simulink model "chart"  (R2025b)
settings: Solver=VariableStepAuto  StartTime=0.0  StopTime=10.0  RelTol=1e-3
undefined symbols (not defined in the file or in its folder): AppAirBtn, AppAmplitude, AppPeriods, AppSharpness, AppZeroBtn, xx, yy
libraries: slrealtimeutilitieslib x7, dspstat3 x2, simulink x1, etargetslib x1, dspmathops x1
settings Model: Creator=Huawei  LastModifiedBy=Huawei

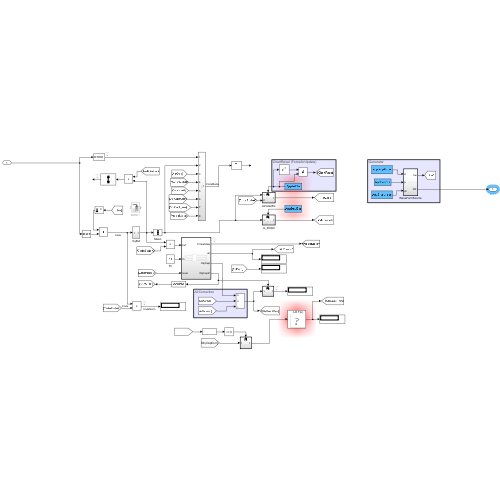
[thumbnail: Simulink's stored preview of the top-level diagram]
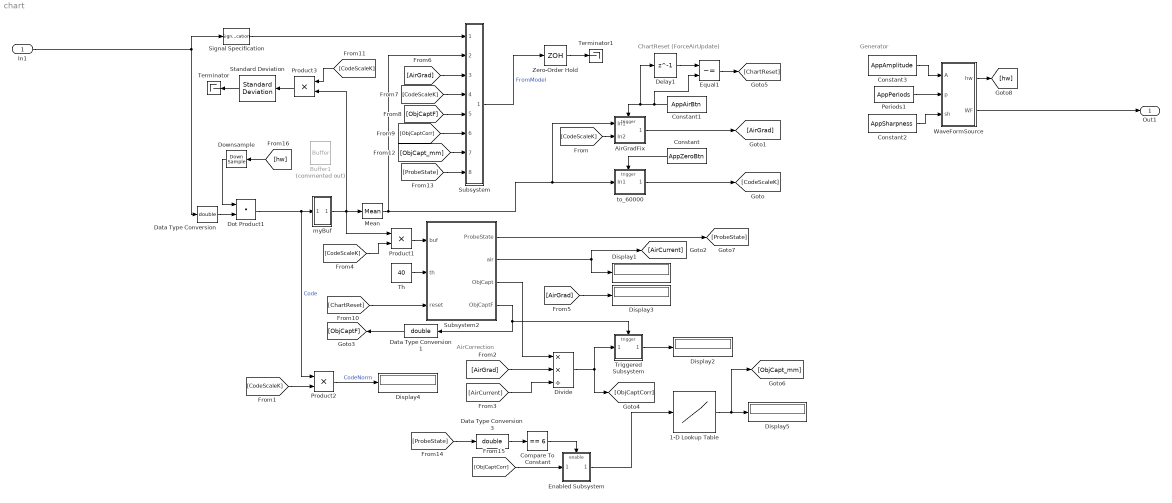
== system chart ==
  note: AirCorrection
  note: ChartReset (ForceAirUpdate)
  note: Generator
  In1 : Inport
  1-D Lookup Table : Lookup_n-D  NumberOfTableDimensions=1  LookupTableObject=myLUTobj  BreakpointsForDimension1=xx  IndexSearchMethod=Linear search  Table=yy  InternalRulePriority=Speed  RndMeth=Simplest
  AirGradFix : Subsystem  TreatAsAtomicUnit=on
  Buffer1 : Buffer  Commented=on  N=8  V=7  OutputFrames=off
  Compare To Constant : simulink/Logic and Bit Operations/Compare To Constant  relop===  const=6  OutDataTypeStr=boolean
  Constant : Constant  Value=AppZeroBtn  OutDataTypeStr=boolean  SampleTime=0.02
  Constant1 : Constant  Value=AppAirBtn  OutDataTypeStr=boolean  SampleTime=0.02
  Constant2 : Constant  Value=AppSharpness  SampleTime=0.02
  Constant3 : Constant  Value=AppAmplitude  SampleTime=0.02
  Data Type Conversion : DataTypeConversion  OutDataTypeStr=double  SaturateOnIntegerOverflow=off  RndMeth=Floor
  Data Type Conversion1 : DataTypeConversion  OutDataTypeStr=double  SaturateOnIntegerOverflow=off  RndMeth=Floor
  Data Type Conversion3 : DataTypeConversion  OutDataTypeStr=double  SaturateOnIntegerOverflow=off  RndMeth=Floor
  Delay1 : Delay  DelayLength=1  InputProcessing=Columns as channels (frame based)
  Display{1..5} (5 alike) : Display
      settings: Format=bank
  Divide : Product  Inputs=**/
  Dot Product1 : DotProduct  OutDataTypeStr=Inherit: Inherit via internal rule
  Downsample : DownSample  N=4
  Enabled Subsystem : Subsystem  TreatAsAtomicUnit=on
  Equal1 : RelationalOperator  Operator=~=  OutDataTypeStr=boolean  RndMeth=Simplest  InputSameDT=off
  Mean : dspstat3/Mean  run=off  InputProcessing=Columns as channels (frame based)  reset_popup=None  directionMode=Each column  dimension=1  roiEnable=off  roiType=Rectangles  roiPortion=Entire ROI  roiOutput=Individual statistics for each ROI  roiFlag=off  roundingMode=Floor  overflowMode=off  outputDataTypeStr=Inherit: Same as accumulator  outputMin=[]  outputMax=[]  outputLastDataTypeStr=Inherit: Same as accumulator
  Periods1 : Constant  Value=AppPeriods  SampleTime=0.02
  Product1 : Product
  Product2 : Product
  Product3 : Product
  Signal Specification : SignalSpecification  Dimensions=5000
  Standard Deviation : dspstat3/Standard Deviation  run=off  directionMode=Each column  dimension=1  InputProcessing=Columns as channels (frame based)  reset_popup=None  roiEnable=off  roiType=Rectangles  roiPortion=Entire ROI  roiOutput=Individual statistics for each ROI  roiFlag=off
  Subsystem : Subsystem
  Subsystem2 : Subsystem  TreatAsAtomicUnit=on  SystemSampleTime=0.02
  Terminator : Terminator
  Terminator1 : Terminator
  Th : Constant  Value=40  SampleTime=0.02
  Triggered Subsystem : Subsystem  TreatAsAtomicUnit=on
  WaveFormSource : Subsystem  TreatAsAtomicUnit=on  SystemSampleTime=0.02
  Zero-Order Hold : ZeroOrderHold  SampleTime=0.02
  myBuf : Subsystem
  to_60000 : Subsystem
  Out1 : Outport
  wires:
  Triggered Subsystem/1(Out1) -> Display2/1
  Data Type Conversion3/1 -> Compare To Constant/1
  [CodeScaleK] -> Product3/1
  Data Type Conversion1/1 -> [ObjCaptF]
  [hw] -> Downsample/1
  myBuf/1(Out1) -> Product3/2, Mean/1, Product1/1
  [CodeScaleK] -> AirGradFix/2(In2)
  Th/1 -> Subsystem2/2(th)
  [CodeScaleK] -> Subsystem/4(In3)
  Compare To Constant/1 -> Enabled Subsystem/Enable
  [ObjCaptCorr] -> Subsystem/6(In6)
  Zero-Order Hold/1 -> Terminator1/1
  Standard Deviation/1 -> Terminator/1
  AirGradFix/1(Out1) -> [AirGrad]
  Subsystem2/3(ObjCapt) -> Divide/1
  Product3/1 -> Standard Deviation/1
  Downsample/1 -> Dot Product1/1
  Dot Product1/1 -> myBuf/1(In1), Product2/1  "Code"
  [AirGrad] -> Display3/1
  Delay1/1 -> Equal1/1
  Subsystem2/1(" ProbeState") -> [ProbeState]
  Divide/1 -> [ObjCaptCorr], Triggered Subsystem/1(In1)
  Subsystem2/4(ObjCaptF) -> Triggered Subsystem/Trigger, Data Type Conversion1/1
  Product2/1 -> Display4/1  "CodeNorm"
  [ProbeState] -> Subsystem/8(In8)
  Signal Specification/1 -> Subsystem/1(In1)
  Enabled Subsystem/1(Out1) -> 1-D Lookup Table/1
  Constant1/1 -> Equal1/2, Delay1/1, AirGradFix/Trigger
  Subsystem2/2(air) -> [AirCurrent], Display1/1
  [AirGrad] -> Divide/2
  Equal1/1 -> [ChartReset]
  [ObjCaptF] -> Subsystem/5(In5)
  [CodeScaleK] -> Product2/2
  Subsystem/1(Out1) -> Zero-Order Hold/1  "FromModel"
  [AirCurrent] -> Divide/3
  Mean/1 -> Subsystem/2(In4), to_60000/1(In1), AirGradFix/1(In1)
  Product1/1 -> Subsystem2/1(buf)
  Data Type Conversion/1 -> Dot Product1/2
  [ObjCaptCorr] -> Enabled Subsystem/1(In1)
  to_60000/1(Out1) -> [CodeScaleK]
  [ChartReset] -> Subsystem2/3(reset)
  [AirGrad] -> Subsystem/3(In2)
  Constant/1 -> to_60000/Trigger
  1-D Lookup Table/1 -> [ObjCapt_mm], Display5/1
  [CodeScaleK] -> Product1/2
  [ProbeState] -> Data Type Conversion3/1
  [ObjCapt_mm] -> Subsystem/7(In7)
  In1/1 -> Signal Specification/1, Data Type Conversion/1
  WaveFormSource/2(WF) -> Out1/1
  Constant2/1 -> WaveFormSource/3(sh)
  Periods1/1 -> WaveFormSource/2(p)
  WaveFormSource/1(hw) -> [hw]
  Constant3/1 -> WaveFormSource/1(A)

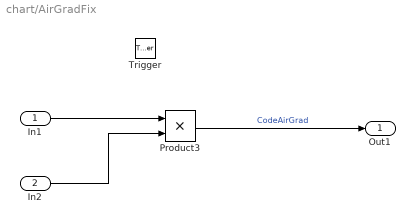
== system chart/AirGradFix ==
  In1 : Inport
  In2 : Inport  Port=2
  Trigger : TriggerPort  TriggerType=either  VariantControl=(inherit)
  Product3 : Product
  Out1 : Outport  InitialOutput=[1]
  wires:
  In1/1 -> Product3/1
  In2/1 -> Product3/2
  Product3/1 -> Out1/1  "CodeAirGrad"

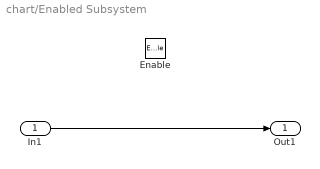
== system chart/Enabled Subsystem ==
  In1 : Inport
  Enable : EnablePort
  Out1 : Outport
  wires:
  In1/1 -> Out1/1

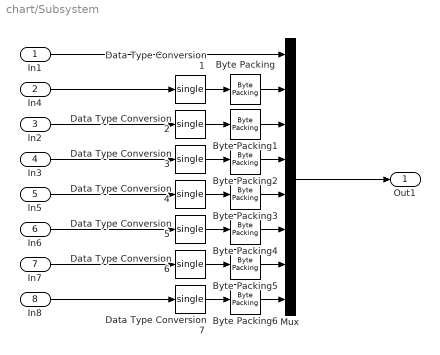
== system chart/Subsystem ==
  In1 : Inport
  In4 : Inport  Port=2
  In2 : Inport  Port=3
  In3 : Inport  Port=4
  In5 : Inport  Port=5
  In6 : Inport  Port=6
  In7 : Inport  Port=7
  In8 : Inport  Port=8
  Byte Packing{,1..6} (7 alike) : slrealtimeutilitieslib/Byte Packing  MaskPackedDataType=uint16  MaskUnpackedDataTypes={'single'}  MaskAlignment=1
  Data Type Conversion{1..7} (7 alike) : DataTypeConversion  OutDataTypeStr=single  SaturateOnIntegerOverflow=off  RndMeth=Floor
  Mux : Mux  Inputs=8
  Out1 : Outport
  wires:
  Byte Packing/1 -> Mux/2
  Data Type Conversion3/1 -> Byte Packing2/1
  Byte Packing1/1 -> Mux/3
  Data Type Conversion1/1 -> Byte Packing/1
  In2/1 -> Data Type Conversion2/1
  Byte Packing2/1 -> Mux/4
  Mux/1 -> Out1/1
  In1/1 -> Mux/1
  Data Type Conversion2/1 -> Byte Packing1/1
  In4/1 -> Data Type Conversion1/1
  In3/1 -> Data Type Conversion3/1
  Data Type Conversion4/1 -> Byte Packing3/1
  In5/1 -> Data Type Conversion4/1
  Byte Packing3/1 -> Mux/5
  Data Type Conversion5/1 -> Byte Packing4/1
  In6/1 -> Data Type Conversion5/1
  Byte Packing4/1 -> Mux/6
  Data Type Conversion6/1 -> Byte Packing5/1
  In7/1 -> Data Type Conversion6/1
  Byte Packing5/1 -> Mux/7
  Data Type Conversion7/1 -> Byte Packing6/1
  In8/1 -> Data Type Conversion7/1
  Byte Packing6/1 -> Mux/8

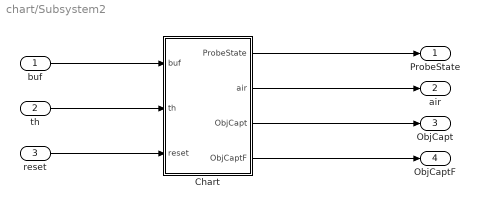
== system chart/Subsystem2 ==
  buf : Inport
  th : Inport  Port=2
  reset : Inport  Port=3
  Chart : Stateflow chart  Tag=myChart  TreatAsAtomicUnit=on  SystemSampleTime=0.02
  " ProbeState" : Outport
  air : Outport  Port=2
  ObjCapt : Outport  Port=3
  ObjCaptF : Outport  Port=4
  wires:
  Chart/4(ObjCaptF) -> ObjCaptF/1
  reset/1 -> Chart/3(reset)
  buf/1 -> Chart/1(buf)
  th/1 -> Chart/2(th)
  Chart/1(" ProbeState") -> " ProbeState"/1
  Chart/2(air) -> air/1
  Chart/3(ObjCapt) -> ObjCapt/1

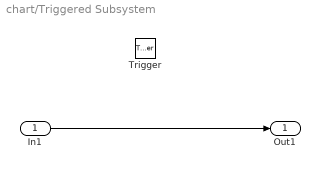
== system chart/Triggered Subsystem ==
  In1 : Inport
  Trigger : TriggerPort  TriggerType=either  VariantControl=(inherit)
  Out1 : Outport
  wires:
  In1/1 -> Out1/1

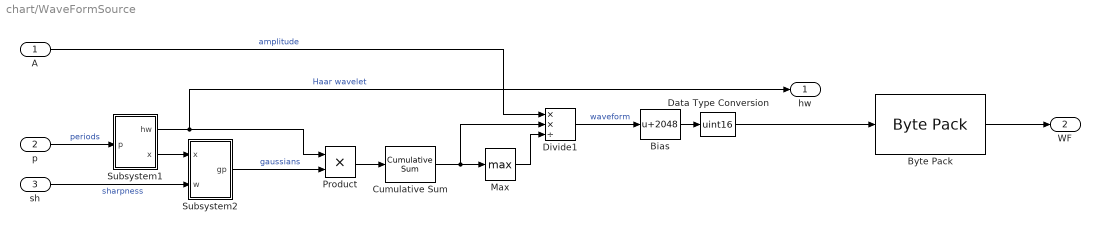
== system chart/WaveFormSource ==
  A : Inport
  p : Inport  Port=2
  sh : Inport  Port=3
  Bias : Bias  Bias=2048  SaturateOnIntegerOverflow=off
  Byte Pack : etargetslib/Byte Pack  datatypes={'uint16'}  byteAlign=1
  Cumulative Sum : dspmathops/Cumulative Sum  dim=Channels (running sum)  InputProcessing=Columns as channels (frame based)  reset_popup=None  roundingMode=Floor  overflowMode=off  outputDataTypeStr=Inherit: Same as accumulator  outputMin=[]  outputMax=[]  outputLastDataTypeStr=Inherit: Same as accumulator
  Data Type Conversion : DataTypeConversion  OutDataTypeStr=uint16  RndMeth=Round  SaturateOnIntegerOverflow=off
  Divide1 : Product  Inputs=**/
  Max : MinMax  Function=max
  Product : Product
  Subsystem1 : Subsystem
  Subsystem2 : Subsystem
  hw : Outport
  WF : Outport  Port=2
  wires:
  Product/1 -> Cumulative Sum/1
  Cumulative Sum/1 -> Divide1/2, Max/1
  Subsystem2/1(gp) -> Product/2  "gaussians"
  Subsystem1/2(x) -> Subsystem2/1(x)
  sh/1 -> Subsystem2/2(w)  "sharpness"
  Subsystem1/1(hw) -> hw/1, Product/1  "Haar wavelet"
  Max/1 -> Divide1/3
  p/1 -> Subsystem1/1(p)  "periods"
  Divide1/1 -> Bias/1  "waveform"
  A/1 -> Divide1/1  "amplitude"
  Bias/1 -> Data Type Conversion/1
  Data Type Conversion/1 -> Byte Pack/1
  Byte Pack/1 -> WF/1

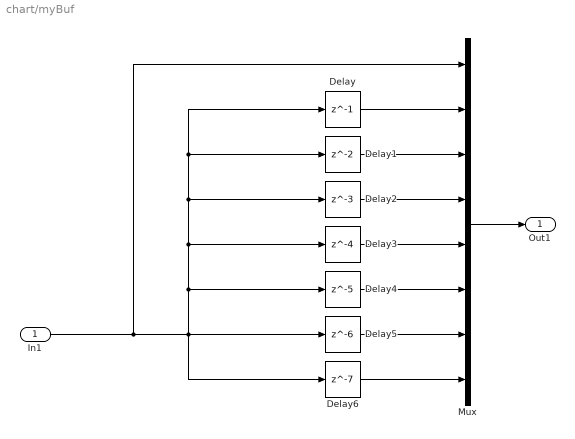
== system chart/myBuf ==
  In1 : Inport
  Delay : Delay  DelayLength=1  InputProcessing=Columns as channels (frame based)
  Delay1 : Delay  InputProcessing=Columns as channels (frame based)
  Delay2 : Delay  DelayLength=3  InputProcessing=Columns as channels (frame based)
  Delay3 : Delay  DelayLength=4  InputProcessing=Columns as channels (frame based)
  Delay4 : Delay  DelayLength=5  InputProcessing=Columns as channels (frame based)
  Delay5 : Delay  DelayLength=6  InputProcessing=Columns as channels (frame based)
  Delay6 : Delay  DelayLength=7  InputProcessing=Columns as channels (frame based)
  Mux : Mux  Inputs=8
  Out1 : Outport
  wires:
  In1/1 -> Mux/1, Delay6/1, Delay4/1, Delay3/1, Delay2/1, Delay1/1, Delay/1, Delay5/1
  Delay/1 -> Mux/2
  Delay1/1 -> Mux/3
  Delay2/1 -> Mux/4
  Delay3/1 -> Mux/5
  Delay4/1 -> Mux/6
  Delay5/1 -> Mux/7
  Delay6/1 -> Mux/8
  Mux/1 -> Out1/1

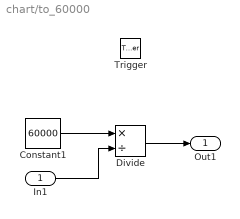
== system chart/to_60000 ==
  In1 : Inport
  Trigger : TriggerPort  TriggerType=either  VariantControl=(inherit)  PortDimensions=1
  Constant1 : Constant  Value=60000  SampleTime=-1
  Divide : Product  Inputs=*/
  Out1 : Outport  InitialOutput=[0.0146]
  wires:
  Constant1/1 -> Divide/1
  In1/1 -> Divide/2
  Divide/1 -> Out1/1

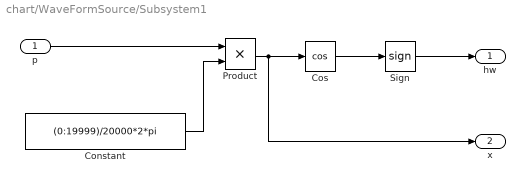
== system chart/WaveFormSource/Subsystem1 ==
  p : Inport
  Constant : Constant  Value=(0:19999)/20000*2*pi
  Cos : Trigonometry  Operator=cos
  Product : Product
  Sign : Signum
  hw : Outport
  x : Outport  Port=2
  wires:
  Cos/1 -> Sign/1
  Product/1 -> x/1, Cos/1
  Constant/1 -> Product/2
  p/1 -> Product/1
  Sign/1 -> hw/1

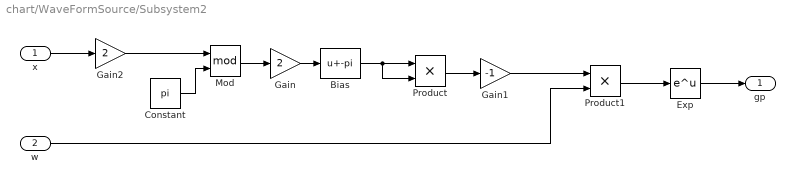
== system chart/WaveFormSource/Subsystem2 ==
  x : Inport
  w : Inport  Port=2
  Bias : Bias  Bias=-pi  SaturateOnIntegerOverflow=off
  Constant : Constant  Value=pi
  Exp : Math
  Gain : Gain  Gain=2
  Gain1 : Gain  Gain=-1
  Gain2 : Gain  Gain=2
  Mod : Math  Operator=mod
  Product : Product
  Product1 : Product
  gp : Outport
  wires:
  x/1 -> Gain2/1
  Constant/1 -> Mod/2
  Mod/1 -> Gain/1
  Gain/1 -> Bias/1
  Bias/1 -> Product/2, Product/1
  Product/1 -> Gain1/1
  Gain1/1 -> Product1/1
  Exp/1 -> gp/1
  Product1/1 -> Exp/1
  w/1 -> Product1/2
  Gain2/1 -> Mod/1

== stateflow chart chart/Subsystem2/Chart ==
  state MainChart
    state pActionEntry [parallel]
      settings: executionOrder=1
      state pcond
        entry:
        dif = 0;
        deviation = 1;
        m = buf(end);
        air_th = m + th;
        InAir = true;
        update = false;
        ObjCapt = 0;
        ObjCaptF = false;
        air = 1;
        during:
        dif = buf(end) - buf(1);
        deviation = std( buf);
        m = mean( buf);
        (default) -> (junction 173)
        pcond -> (junction 173)
        (junction 173) -> (junction 175) [order 1] : [m < air_th]
        (junction 173) -> (junction 195) [order 2] : {InAir = false;}
        (junction 175) -> (junction 177) : {InAir = true;}
        (junction 177) -> (junction 195)
        (junction 195) -> (junction 1)
        (junction 1) -> (junction 3) [order 1] : [dif > th]
        (junction 1) -> (junction 19) [order 2]
        (junction 3) -> (junction 6) : { action = down;}
        (junction 19) -> (junction 8) [order 1] : [dif <  -th]
        (junction 19) -> (junction 21) [order 2]
        (junction 8) -> (junction 10) : { action = up;}
        (junction 21) -> (junction 12) [order 1] : [ deviation <= 10]
        (junction 21) -> (junction 23) [order 2] : {action = uncertain;}
        (junction 12) -> (junction 146) : {action = stop;}
        (junction 146) -> (junction 151) [order 1] : [deviation <= 3]
        (junction 146) -> (junction 199) [order 2] : {update = false;}
        (junction 151) -> (junction 155) : {update = true;}
        (junction 155) -> (junction 199)
        (junction 199) -> (junction 202)
        (junction 23) -> (junction 202)
        (junction 10) -> (junction 202)
        (junction 202) -> (junction 241)
        (junction 6) -> (junction 241)
      (default) -> pcond
    state pState [parallel]
      settings: executionOrder=2
      state Air
        state AirUpdate
          entry, during:
          air_th = m + th;
          air = m;
        state UnsteadyAir
        (default) -> UnsteadyAir
        UnsteadyAir -> AirUpdate : [update]
        AirUpdate -> UnsteadyAir : [~update]
      state ToAir
      state ToObject
      state Object
        state ObjectUpdate
          (default) -> (junction 212)
          ObjectUpdate -> (junction 212) [order 1]
          (junction 212) -> (junction 214) [order 1] : [WasInAir]
          (junction 212) -> (junction 218) [order 2]
          (junction 214) -> (junction 216) : {ObjCaptF = ~ObjCaptF;}
          (junction 216) -> (junction 218)
          (junction 218) -> (junction 221) : {ObjCapt = m; WasInAir = false;}
        state UnsteadyObject
        (default) -> UnsteadyObject
        ObjectUpdate -> UnsteadyObject [order 1] : [~update]
        UnsteadyObject -> ObjectUpdate : [update]
      (default) -> Air
      ToAir -> Air [order 2] : [action == stop && InAir]
      Air -> ToObject : [action == down]
          | {WasInAir = true;}
      ToObject -> ToAir [order 1] : [action == up]
      ToAir -> ToObject [order 1] : [action == down]
      Object -> ToAir : [action == up]
      ToAir -> Object [order 3] : [action == stop && ~InAir]
      ToObject -> Object [order 2] : [action == stop]
  (default) -> MainChart
  MainChart -> MainChart : [reset]
  data: buf input; th input; down constant double =1; up constant double =-1; stop constant double =0; action local; ProbeState output Enum: pStateModeType; deviation local; dif local; m local; air_th local; air output; uncertain constant double =2; InAir local; update local; WasInAir local; ObjCapt output; ObjCaptF output; reset input
